simulink model "projets5"  (R2022b)
settings: Solver=FixedStepAuto  StartTime=0.0  StopTime=10.0  RelTol=1e-3  EnableMultiTasking=on
undefined symbols (not defined in the file or in its folder): hw
libraries: raspberrypiAVlib x2
settings Model: SimulationMode=external  Creator=tatan  LastModifiedBy=tatan
settings SolverCC: PositivePriorityOrder=on
settings OptimizationCC: EnhancedBackFolding=on  PassReuseOutputArgsAs=Individual arguments  ZeroExternalMemoryAtStartup=off  ZeroInternalMemoryAtStartup=off  MaxStackSize=64  OptimizeBlockOrder=speed  DifferentSizesBufferReuse=on  OptimizationCustomize=off  EfficientTunableParamExpr=on
settings DebuggingCC: ParameterTunabilityLossMsg=error
settings HardwareCC: ProdBitPerPointer=32  ProdBitPerSizeT=32  ProdBitPerPtrDiffT=32  ProdLargestAtomicInteger=Long  ProdLargestAtomicFloat=Double  ProdWordSize=32  ProdLongLongMode=on  ProdHWDeviceType=ARM Compatible->ARM Cortex  UseEmbeddedCoderFeatures=off  UseSimulinkCoderFeatures=off
settings SFSimCC: SimTargetLang=C++
settings RTWCC: Description=Embedded Coder  SystemTargetFile=ert.tlc  HardwareBoard=Raspberry Pi  TemplateMakefile=ert_default_tmf  RTWVerbose=off  Toolchain=GNU GCC Embedded Linux  BuildConfiguration=Faster Runs
settings CodeAppCC: ForceParamTrailComments=on  OperatorAnnotations=on  SimulinkDataObjDesc=on  SFDataObjDesc=on  InsertBlockDesc=on
settings ERTTargetCC: SupportNonInlinedSFcns=on  SupportVariableSizeSignals=on  ExtMode=on  ExtModeTransport=2  ExtModeStaticAlloc=on  ExtModeMexFile=ext_xcp  ExtModeMexArgs='192.168.43.177' 0 17725  ExtModeIntrfLevel=Level2 - Open  ERTSrcFileBannerTemplate=codertarget_code_template.cgt  ERTHdrFileBannerTemplate=codertarget_code_template.cgt  ERTDataSrcFileTemplate=codertarget_code_template.cgt  ERTDataHdrFileTemplate=codertarget_code_template.cgt

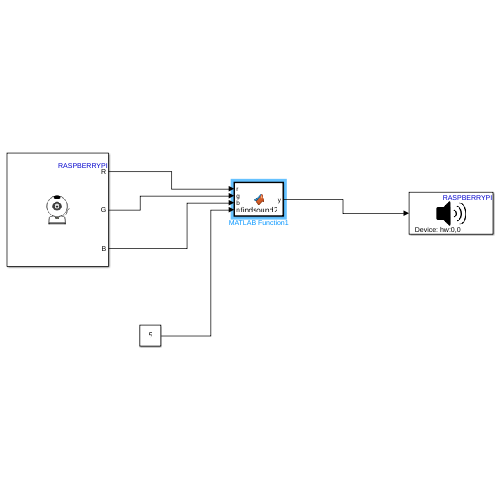
[thumbnail: Simulink's stored preview of the top-level diagram]
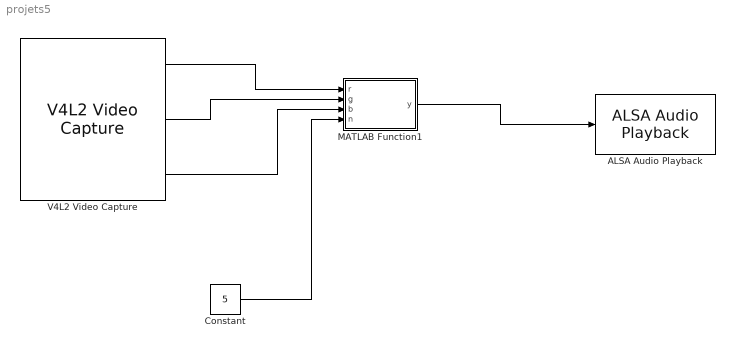
== system projets5 ==
  ALSA Audio Playback : raspberrypiAVlib/ALSA Audio Playback  deviceStr=hw:0,0  sampleRateEnum=44100  queueDuration=0.5  blockPlatform=LINUX
  Constant : Constant  Value=5
  MATLAB Function1 : MATLAB Function  TreatAsAtomicUnit=on
  V4L2 Video Capture : raspberrypiAVlib/V4L2 Video Capture  DeviceName=/dev/video0  Resolution=160x120  CustomResolution=[ 320, 240 ]  PixelFormat=RGB  SampleTime=1  pixelOrder=planar  simOutput=Colorbars  imSizeSelection=320x240  imSize=[640, 480]  roi=[0, 0, 640, 480]  m_devName='/dev/video0'  blockPlatform=LINUX  HorizontalFlip=off  VerticalFlip=off  Brightness=0.5  Saturation=0.5  Contrast=0.5  Sharpness=0.5  CameraPan=0  CameraTilt=0  CameraZoom=0.5  EnableManualFocus=on  ManualFocus=0.5
  wires:
  V4L2 Video Capture/1 -> MATLAB Function1/1(r)
  V4L2 Video Capture/2 -> MATLAB Function1/2(g)
  V4L2 Video Capture/3 -> MATLAB Function1/3(b)
  Constant/1 -> MATLAB Function1/4(n)
  MATLAB Function1/1(y) -> ALSA Audio Playback/1

== matlab function projets5/MATLAB Function1 ==
  data: r input; y output; g input; b input; n input
function y =findsound2(r,g,b,n)
    s = size(r);
    rgb = zeros(s(1,1),s(1,2),3);
    for l=1:s(1,1)
        for c=1:s(1,2)
            rgb(l,c,:) = [r(l,c) g(l,c) b(l,c)];
        end
    end
    angle = trouverAngle(rgb, n);
    w = pulsation(angle(1));
    %t = linspace(0,10,10*int16(2*w));
    t= linspace(0,10,100000);
    y = int16(transpose(amplitude(angle(1)) * sin(w*t)));
end

function amp = amplitude(angle)
    amp = abs(angle(1)/90);
end

function w = pulsation(angle)
    w = 440 + (angle / 90) * 220;
end

function angle = trouverAngle(img, n)
    i = findcolor(img,n);
    [img,map] = quantize(img,n);
    imshow(img,map);
    coef = regressionlineair(img, i);
    surete = coef(1,3);
    coef = coef(1,2);
    coef = 1/coef;
    angle = [-mod(atan(coef)*360/(2*pi),180)+90, surete ];
    %angle = atan(coef)*360/(2*pi)
end

function icol = findcolor(img,n)
    [img,map] = quantize(img,n);
    index=0;
    minerror = regressionlineair(img,index);
    minerror = minerror(1,3);
    for i=1:n-1
        therror = regressionlineair(img,i);
        therror = therror(1,3);
        if therror<minerror
            minerror = therror;
            index = i;
        end
    end
    icol = index;
end

function coef = regressionlineair(img, i)
    S = size(img);
    Points = [];
    for l=1:S(1,1)
       Points = [ Points trouvermilieux(img,l,i)];
    end
    x = Points(1,:);
    x = transpose(x);
    s = size(x);
    un = ones(s(1,1),1);
    %x = [un x];
    y = Points(2,:);
    y = transpose(y);
    x = double(x);
    y = double(y);
    %[b, bint, r, rint, stats] = regress(y,x);
    [p,S] = polyfit(x,y,1);
    [y_fit,delta] = polyval(p,x,S);
    %stats
    %autcoef = regress(y,xe)
    %coef = x\y
    b = [p mean(delta)];
    coef = b;
    %coef = 1
end


function pix = trouvermilieux(img, l, i)
    S = size(img);
    c = 1;
    temp = [];
    while c<S(1,2)
        while img(l,c)~=i & c < S(1,2)
            c=c+1;
        end

        debut = c;
        while img(l,c)==i & c < S(1,2)
            c=c+1;
        end
        fin = int16(c-1);
        if img(l,debut)==i & img(l,fin)==i
            vec = [l int16((debut+fin)/2)];
            vec = transpose(vec);
            temp = [ temp vec];
        end
    end
    pix = temp;
end

function [img,map] = quantize(rgb,k)
    S=size(rgb);
    tmp = ones(3,S(1,1)*S(1,2));
    for l=1:S(1,1)
        tmp(:,(l-1)*S(1,2)+1:l*S(1,2))=transpose(squeeze(rgb(l,:,:)));
    end
    [idx,C] = kmeans(transpose(tmp),k);
    imgt = ones(S(1,1)+1,S(1,2));
    for i=1:S(1,1)*S(1,2)
        imgt(uint32(i/S(1,2))+1,mod(i,S(1,2))+1) = idx(i);
%           if idx(i)==0
%                idx(i)
%           end
    end
    imgt(S(1,1)+1,:) = [];

    imgt = medfilt2(imgt,[5,5]);
    img = imgt;
    map = uint8(C);
end
